simulink model "test_attitude"  (R2017a)
settings: Solver=VariableStepAuto  StartTime=0.0  StopTime=10.0  FixedStep=0.01  RelTol=1e-3
settings Model: Creator=aditya  LastModifiedBy=aditya

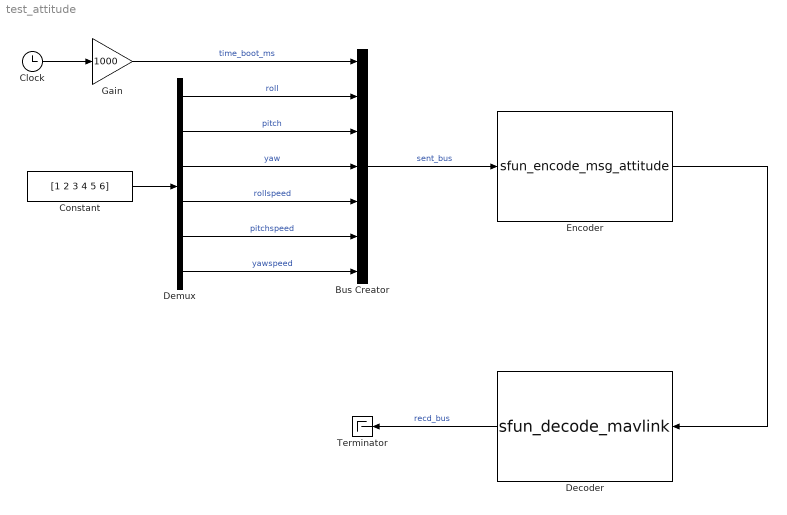
== system test_attitude ==
  Bus Creator : BusCreator  Inputs=7  OutDataTypeStr=Bus: mavlink_attitude_t  NonVirtualBus=on
  Clock : Clock
  Constant : Constant  Value=[1 2 3 4 5 6]  OutDataTypeStr=single
  Decoder : S-Function  FunctionName=sfun_decode_mavlink  SFunctionDeploymentMode=off  EnableBusSupport=off
  Demux : Demux  Outputs=6
  Encoder : S-Function  FunctionName=sfun_encode_msg_attitude  SFunctionDeploymentMode=off  EnableBusSupport=off
  Gain : Gain  Gain=1000  OutDataTypeStr=uint32
  Terminator : Terminator
  wires:
  Encoder/1 -> Decoder/1
  Bus Creator/1 -> Encoder/1  "sent_bus"
  Clock/1 -> Gain/1
  Gain/1 -> Bus Creator/1  "time_boot_ms"
  Demux/6 -> Bus Creator/7  "yawspeed"
  Demux/5 -> Bus Creator/6  "pitchspeed"
  Demux/4 -> Bus Creator/5  "rollspeed"
  Demux/3 -> Bus Creator/4  "yaw"
  Demux/2 -> Bus Creator/3  "pitch"
  Demux/1 -> Bus Creator/2  "roll"
  Constant/1 -> Demux/1
  Decoder/1 -> Terminator/1  "recd_bus"
